simulink model "model_dyskretny_2_reg"  (R2020a)
settings: Solver=VariableStepAuto  StartTime=0.0  StopTime=10.0  RelTol=1e-3
values from neighbouring files (symbols this model uses):
  K = acker(A,B, [zb1, zb2, zb3])    [zad1_10.m]    (also in zad1_6.m = [k1 k2 k3]; zad1_6_1.m = acker(A,B, [zb(3), zb(3), zb(3)]); zad1_6_2.m = acker(A,B, [zb1, complex(a(1), b(3)), complex(a(1), -b(3))]); zad1_9.m)
  T = 0.5    [pom.m]    (also in zad1_10.m; zad1_4.m; zad1_6_1.m; zad1_6_2.m)
settings Model: Creator=jakub  LastModifiedBy=jakub

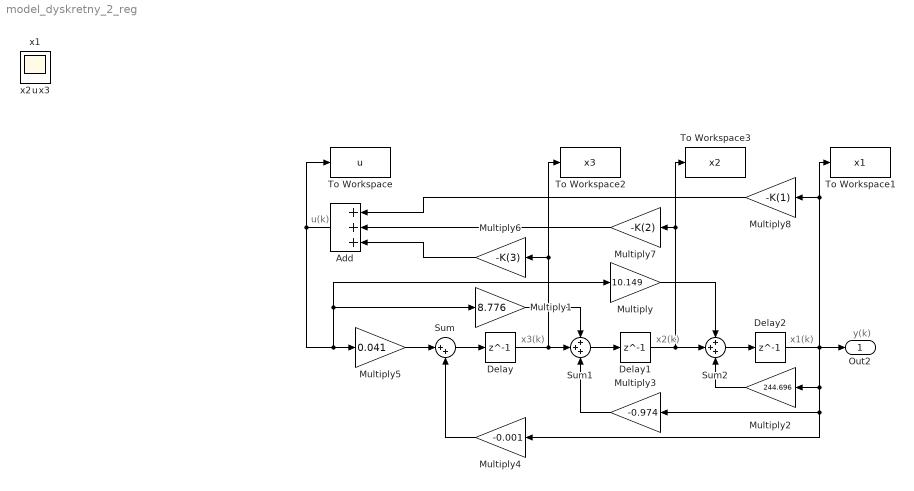
== system model_dyskretny_2_reg ==
  note: y(k)
  note: u(k)
  note: x2(k)
  note: x3(k)
  note: x1(k)
  Add : Sum  Inputs=+++
  Delay : Delay  DelayLength=1  InitialCondition=5  SampleTime=T
  Delay1 : Delay  DelayLength=1  InitialCondition=-2  SampleTime=T
  Delay2 : Delay  DelayLength=1  InitialCondition=-1  SampleTime=T
  Multiply : Gain  Gain=10.149
  Multiply1 : Gain  Gain=8.776
  Multiply2 : Gain  Gain=244.696
  Multiply3 : Gain  Gain=-0.974
  Multiply4 : Gain  Gain=-0.001
  Multiply5 : Gain  Gain=0.041
  Multiply6 : Gain  Gain=-K(3)
  Multiply7 : Gain  Gain=-K(2)
  Multiply8 : Gain  Gain=-K(1)
  Sum : Sum  Inputs=|++
  Sum1 : Sum  Inputs=+++
  Sum2 : Sum  Inputs=+++
  To Workspace : ToWorkspace  VariableName=u  SaveFormat=Structure With Time  SampleTime=-1
  To Workspace1 : ToWorkspace  VariableName=x1  SaveFormat=Structure With Time  SampleTime=-1
  To Workspace2 : ToWorkspace  VariableName=x3  SaveFormat=Structure With Time  SampleTime=-1
  To Workspace3 : ToWorkspace  VariableName=x2  SaveFormat=Structure With Time  SampleTime=-1
  Out2 : Outport
  u : Scope
  x1 : Scope
  x2 : Scope
  x3 : Scope
  wires:
  Add/1 -> To Workspace/1, Multiply/1, Multiply1/1, Multiply5/1
  Sum/1 -> Delay/1
  Multiply5/1 -> Sum/1
  Sum1/1 -> Delay1/1
  Delay1/1 -> To Workspace3/1, Multiply7/1, Sum2/2
  Sum2/1 -> Delay2/1
  Delay/1 -> To Workspace2/1, Multiply6/1, Sum1/2
  Delay2/1 -> To Workspace1/1, Multiply8/1, Out2/1, Multiply4/1, Multiply3/1, Multiply2/1
  Multiply1/1 -> Sum1/1
  Multiply/1 -> Sum2/1
  Multiply3/1 -> Sum1/3
  Multiply4/1 -> Sum/2
  Multiply2/1 -> Sum2/3
  Multiply8/1 -> Add/1
  Multiply7/1 -> Add/2
  Multiply6/1 -> Add/3
